simulink model "sig_kadet"  (R2024a)
settings: Solver=FixedStepAuto  StartTime=0.0  StopTime=10.0  FixedStep=framePeriod_s  RelTol=1e-3
undefined symbols (not defined in the file): Control, DiscIntNeverNeededParam, framePeriod_s
libraries: aerolibconvert2 x7, slpidlib x6
(part 1 of 2)
settings Model: Creator=brian  LastModifiedBy=zchen
settings SolverCC: AlgebraicLoopSolver=TrustRegion
settings OptimizationCC: DefaultParameterBehavior=Inlined  GainParamInheritBuiltInType=on  UseFloatMulNetSlope=on  DefaultUnderspecifiedDataType=single  InlineInvariantSignals=on  PassReuseOutputArgsAs=Individual arguments  ZeroExternalMemoryAtStartup=off  ZeroInternalMemoryAtStartup=off  NoFixptDivByZeroProtection=on  EfficientFloat2IntCast=on  LifeSpan=1  OptimizeBlockOrder=speed  DifferentSizesBufferReuse=on  EfficientTunableParamExpr=on
settings DebuggingCC: ParameterTunabilityLossMsg=error  UnconnectedInputMsg=warning  UnconnectedOutputMsg=warning  UnconnectedLineMsg=warning
settings HardwareCC: ProdBitPerPointer=32  ProdBitPerSizeT=32  ProdBitPerPtrDiffT=32  ProdLargestAtomicInteger=Long  ProdLargestAtomicFloat=Double  ProdWordSize=32  ProdLongLongMode=on  ProdHWDeviceType=NXP->Cortex-M4
settings ModelReferenceCC: EnableRefExpFcnMdlSchedulingChecks=on  ModelReferenceNumInstancesAllowed=Single
settings SFSimCC: SimParseCustomCode=off  MATLABDynamicMemAlloc=off
settings RTWCC: Description=Embedded Coder  SystemTargetFile=ert.tlc  GenCodeOnly=on  TemplateMakefile=ert_default_tmf  RTWVerbose=off  BuildConfiguration=Faster Runs  TargetLang=C++  GPUComputeCapability=3.5  DLArmComputeVersion=19.05
settings CodeAppCC: ForceParamTrailComments=on  IgnoreCustomStorageClasses=off  OperatorAnnotations=on  SimulinkDataObjDesc=on  SFDataObjDesc=on  CustomSymbolStrGlobalVar=rt$N$M  CustomSymbolStrType=$N$M  CustomSymbolStrFcn=$N$M$F  CustomSymbolStrMacro=$N$M  InsertBlockDesc=on
settings ERTTargetCC: TargetLangStandard=C++03 (ISO)  IncludeMdlTerminateFcn=off  CombineSignalStateStructs=on  SuppressErrorStatus=on  SupportAbsoluteTime=off  CodeInterfacePackaging=C++ class  SupportNonFinite=off  SupportComplex=off  ERTHeaderFileRootName=autocode$E  ERTSourceFileRootName=autocode$E  InlinedParameterPlacement=NonHierarchical  RootIOFormat=Structure reference  ERTCustomFileTemplate=example_file_process.tlc  ERTFilePackagingFormat=Compact  ArrayContainerType=std::array

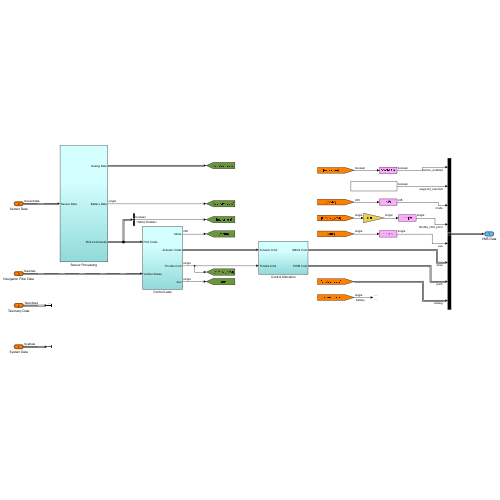
[thumbnail: Simulink's stored preview of the top-level diagram]
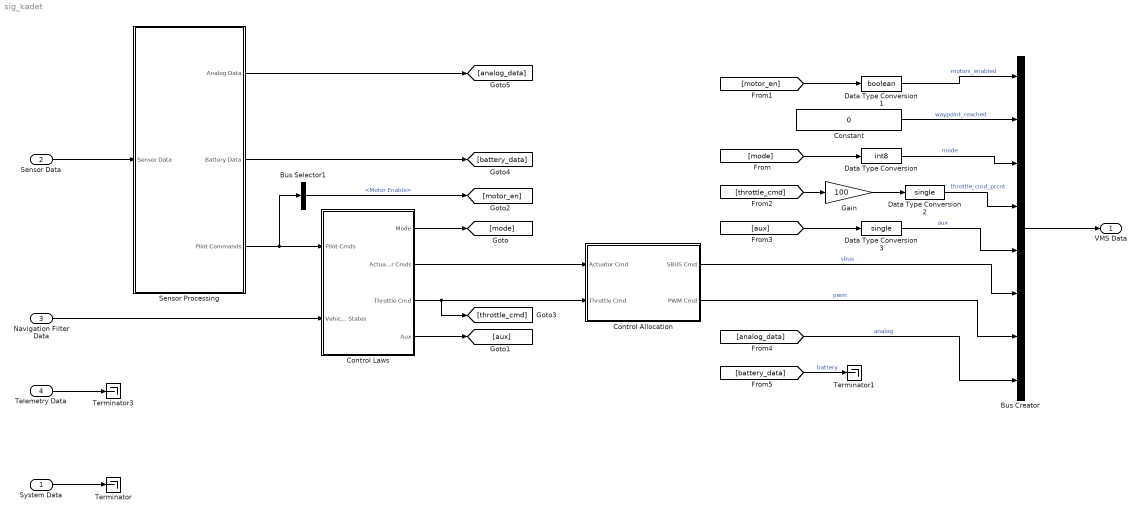
== system sig_kadet ==
  System Data : Inport  OutDataTypeStr=Bus: SysData  SampleTime=framePeriod_s  BusOutputAsStruct=on
  Sensor Data : Inport  Port=2  OutDataTypeStr=Bus: SensorData  SampleTime=framePeriod_s  BusOutputAsStruct=on
  Navigation Filter Data : Inport  Port=3  OutDataTypeStr=Bus: NavData  SampleTime=framePeriod_s  BusOutputAsStruct=on
  Telemetry Data : Inport  Port=4  OutDataTypeStr=Bus: TelemData  SampleTime=framePeriod_s  BusOutputAsStruct=on
  Bus Creator : BusCreator  Inputs=8
  Bus Selector1 : BusSelector  OutputSignals=Motor Enable
  Constant : Constant  Value=0  OutDataTypeStr=boolean
  Control Allocation : Subsystem
  Control Laws : Subsystem
  Data Type Conversion : DataTypeConversion  OutDataTypeStr=int8  SaturateOnIntegerOverflow=off  RndMeth=Floor
  Data Type Conversion1 : DataTypeConversion  OutDataTypeStr=boolean  SaturateOnIntegerOverflow=off  RndMeth=Floor
  Data Type Conversion2 : DataTypeConversion  OutDataTypeStr=single  SaturateOnIntegerOverflow=off  RndMeth=Floor
  Data Type Conversion3 : DataTypeConversion  OutDataTypeStr=single  SaturateOnIntegerOverflow=off  RndMeth=Floor
  Gain : Gain  Gain=100  OutDataTypeStr=single
  Sensor Processing : Subsystem
  Terminator : Terminator
  Terminator1 : Terminator
  Terminator3 : Terminator
  VMS Data : Outport  OutDataTypeStr=Bus: VmsData  SampleTime=framePeriod_s  BusOutputAsStruct=on
  wires:
  System Data/1 -> Terminator/1
  Sensor Data/1 -> Sensor Processing/1(Sensor Data)
  Telemetry Data/1 -> Terminator3/1
  Navigation Filter Data/1 -> Control Laws/2(Vehicle States)
  Control Laws/1(Mode) -> [mode]
  Control Laws/4(Aux) -> [aux]
  [mode] -> Data Type Conversion/1
  Data Type Conversion/1 -> Bus Creator/3  "mode"
  Bus Selector1/1 -> [motor_en]  "<Motor Enable>"
  [motor_en] -> Data Type Conversion1/1
  Data Type Conversion1/1 -> Bus Creator/1  "motors_enabled"
  Constant/1 -> Bus Creator/2  "waypoint_reached"
  Control Laws/3(Throttle Cmd) -> Control Allocation/2(Throttle Cmd), [throttle_cmd]
  [throttle_cmd] -> Gain/1
  Gain/1 -> Data Type Conversion2/1
  Data Type Conversion2/1 -> Bus Creator/4  "throttle_cmd_prcnt"
  [aux] -> Data Type Conversion3/1
  Data Type Conversion3/1 -> Bus Creator/5  "aux"
  Bus Creator/1 -> VMS Data/1
  Sensor Processing/3(Pilot Commands) -> Bus Selector1/1, Control Laws/1(Pilot Cmds)
  Sensor Processing/2(Battery Data) -> [battery_data]
  Sensor Processing/1(Analog Data) -> [analog_data]
  [analog_data] -> Bus Creator/8  "analog"
  Control Laws/2(Actuator Cmds) -> Control Allocation/1(Actuator Cmd)
  Control Allocation/1(SBUS Cmd) -> Bus Creator/6  "sbus"
  Control Allocation/2(PWM Cmd) -> Bus Creator/7  "pwm"
  [battery_data] -> Terminator1/1  "battery"

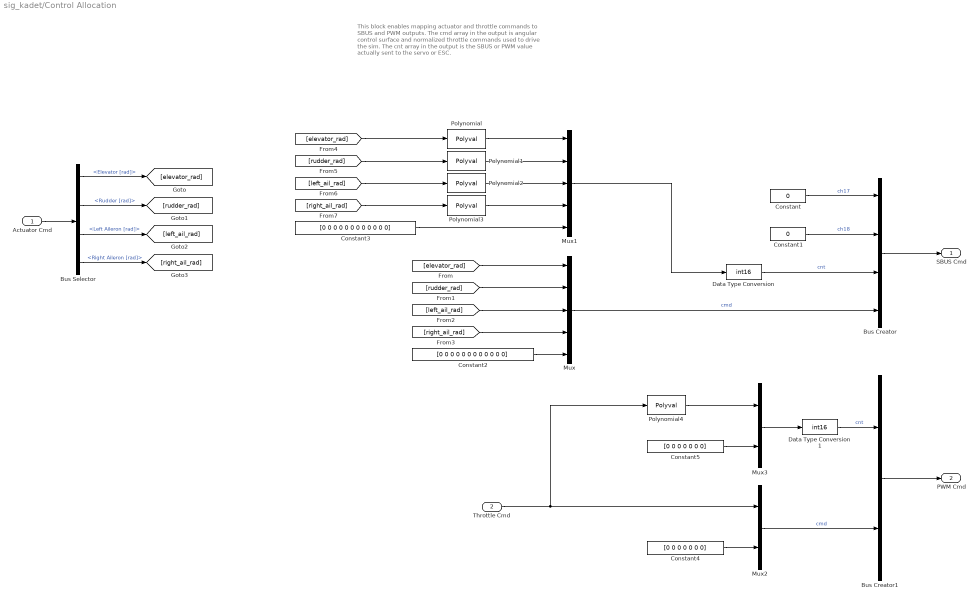
== system sig_kadet/Control Allocation ==
  note: This block enables mapping actuator and throttle commands
      | to SBUS and PWM outputs. The cmd array in the output
      | is angular control surface and normalized throttle commands
      | used to drive the sim. The cnt array in the output is the SBUS
      | or PWM value actually sent to the servo or ESC.
  Actuator Cmd : Inport
  Throttle Cmd : Inport  Port=2
  Bus Creator : BusCreator  Inputs=4
  Bus Creator1 : BusCreator  Inputs=2
  Bus Selector : BusSelector  OutputSignals=Elevator [rad],Rudder [rad],Left Aileron [rad],Right Aileron [rad]
  Constant : Constant  Value=0  OutDataTypeStr=boolean
  Constant1 : Constant  Value=0  OutDataTypeStr=boolean
  Constant2 : Constant  Value=[0 0 0 0 0 0 0 0 0 0 0 0]  OutDataTypeStr=single
  Constant3 : Constant  Value=[0 0 0 0 0 0 0 0 0 0 0 0]  OutDataTypeStr=single
  Constant4 : Constant  Value=[0 0 0 0 0 0 0]  OutDataTypeStr=single
  Constant5 : Constant  Value=[0 0 0 0 0 0 0]  OutDataTypeStr=single
  Data Type Conversion : DataTypeConversion  OutDataTypeStr=int16  SaturateOnIntegerOverflow=off  RndMeth=Floor
  Data Type Conversion1 : DataTypeConversion  OutDataTypeStr=int16  SaturateOnIntegerOverflow=off  RndMeth=Floor
  Mux : Mux  Inputs=5
  Mux1 : Mux  Inputs=5
  Mux2 : Mux  Inputs=2
  Mux3 : Mux  Inputs=2
  Polynomial : Polyval  Coefs=[1144.32190165984, 167.225360182927, 1558.74885501875, 1026.6382652891]
  Polynomial1 : Polyval  Coefs=[-930.322085258545, 148.612787752928, -1476.11502090935, 1006.01614399429]
  Polynomial2 : Polyval  Coefs=[1097.27825386315, 173.191562145482, 1642.60230905023, 1054.30469578325]
  Polynomial3 : Polyval  Coefs=[930.582953971947, 132.665450728095, 1620.14796233637, 1011.10438715363]
  Polynomial4 : Polyval  Coefs=[1000, 1000]
  SBUS Cmd : Outport
  PWM Cmd : Outport  Port=2
  wires:
  Constant/1 -> Bus Creator/1  "ch17"
  Constant1/1 -> Bus Creator/2  "ch18"
  Bus Creator/1 -> SBUS Cmd/1
  Mux/1 -> Bus Creator/4  "cmd"
  Mux1/1 -> Data Type Conversion/1
  Actuator Cmd/1 -> Bus Selector/1
  Bus Selector/1 -> [elevator_rad]  "<Elevator [rad]>"
  Bus Selector/2 -> [rudder_rad]  "<Rudder [rad]>"
  Bus Selector/3 -> [left_ail_rad]  "<Left Aileron [rad]>"
  Bus Selector/4 -> [right_ail_rad]  "<Right Aileron [rad]>"
  [elevator_rad] -> Mux/1
  [rudder_rad] -> Mux/2
  [left_ail_rad] -> Mux/3
  [right_ail_rad] -> Mux/4
  Constant2/1 -> Mux/5
  Constant3/1 -> Mux1/5
  [right_ail_rad] -> Polynomial3/1
  [left_ail_rad] -> Polynomial2/1
  [rudder_rad] -> Polynomial1/1
  [elevator_rad] -> Polynomial/1
  Data Type Conversion/1 -> Bus Creator/3  "cnt"
  Polynomial/1 -> Mux1/1
  Polynomial1/1 -> Mux1/2
  Polynomial2/1 -> Mux1/3
  Polynomial3/1 -> Mux1/4
  Bus Creator1/1 -> PWM Cmd/1
  Mux2/1 -> Bus Creator1/2  "cmd"
  Constant4/1 -> Mux2/2
  Throttle Cmd/1 -> Polynomial4/1, Mux2/1
  Polynomial4/1 -> Mux3/1
  Constant5/1 -> Mux3/2
  Mux3/1 -> Data Type Conversion1/1
  Data Type Conversion1/1 -> Bus Creator1/1  "cnt"

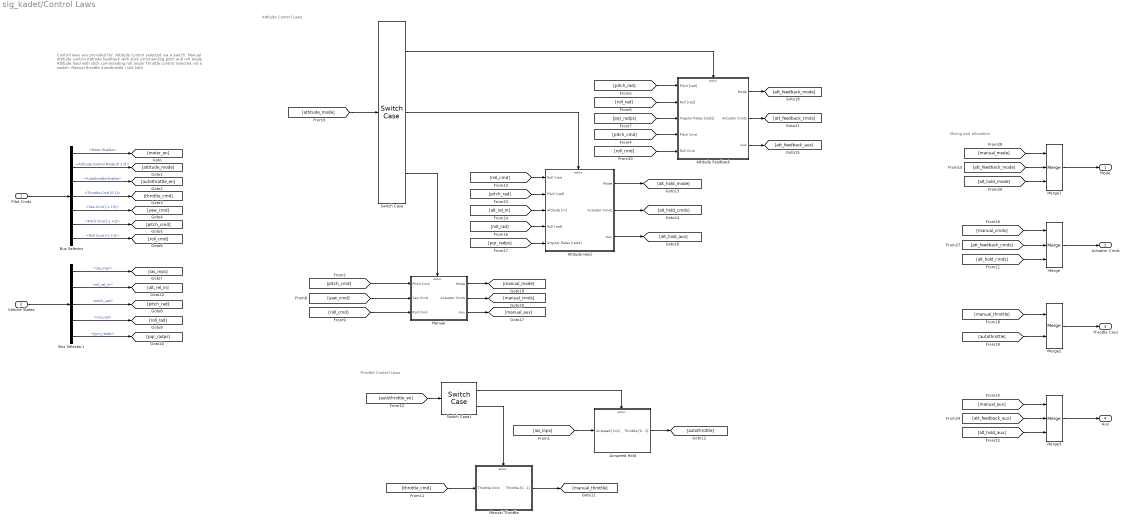
== system sig_kadet/Control Laws ==
  note: Control laws are provided for:
      | Attitude control selected via a switch:
      | Manual attitude control
      | Attitude feedback with stick commanding pitch and roll angle
      | Altitude hold with stick commanding roll angle
      | Throttle control selected via a switch:
      | Manual throttle
      | Autothrottle / IAS hold
  note: Throttle Control Laws
  note: Attitude Control Laws
  note: Mixing and Allocation
  Pilot Cmds : Inport
  Vehicle States : Inport  Port=2
  Airspeed Hold : Subsystem  TreatAsAtomicUnit=on
  Altitude Hold : Subsystem  TreatAsAtomicUnit=on
  Attitude Feedback : Subsystem  TreatAsAtomicUnit=on
  Bus Selector : BusSelector  OutputSignals=Motor Enable,Attitude Control Mode [0 1 2],Autothrottle Enable,Throttle Cmd [0 1],Yaw Cmd [-1 +1],Pitch Cmd [-1 +1],Roll Cmd [-1 +1]
  Bus Selector1 : BusSelector  OutputSignals=ias_mps,alt_rel_m,pitch_rad,roll_rad,gyro_radps
  Manual : Subsystem  TreatAsAtomicUnit=on
  Manual Throttle : Subsystem  TreatAsAtomicUnit=on
  Merge : Merge  Inputs=3
  Merge1 : Merge  Inputs=3
  Merge2 : Merge
  Merge3 : Merge  Inputs=3
  Switch Case : SwitchCase  CaseConditions={1, 2}
  Switch Case1 : SwitchCase
  Mode : Outport
  Actuator Cmds : Outport  Port=2
  Throttle Cmd : Outport  Port=3
  Aux : Outport  Port=4
  wires:
  Pilot Cmds/1 -> Bus Selector/1
  Bus Selector/1 -> [motor_en]  "<Motor Enable>"
  Bus Selector/2 -> [attitude_mode]  "<Attitude Control Mode [0 1 2]>"
  Bus Selector/3 -> [autothrottle_en]  "<Autothrottle Enable>"
  Bus Selector/4 -> [throttle_cmd]  "<Throttle Cmd [0 1]>"
  Bus Selector/5 -> [yaw_cmd]  "<Yaw Cmd [-1 +1]>"
  Bus Selector/6 -> [pitch_cmd]  "<Pitch Cmd [-1 +1]>"
  Bus Selector/7 -> [roll_cmd]  "<Roll Cmd [-1 +1]>"
  Vehicle States/1 -> Bus Selector1/1
  Bus Selector1/1 -> [ias_mps]  "<ias_mps>"
  Bus Selector1/3 -> [pitch_rad]  "<pitch_rad>"
  Bus Selector1/4 -> [roll_rad]  "<roll_rad>"
  Bus Selector1/5 -> [pqr_radps]  "<gyro_radps>"
  Airspeed Hold/1(Throttle [0 - 1]) -> [autothrottle]
  [ias_mps] -> Airspeed Hold/1(Airspeed [m/s])
  [autothrottle_en] -> Switch Case1/1
  [throttle_cmd] -> Manual Throttle/1(Throttle Cmd)
  Switch Case1/1 -> Airspeed Hold/Action
  Switch Case1/2 -> Manual Throttle/Action
  Manual Throttle/1(Throttle [0 - 1]) -> [manual_throttle]
  Manual/1(Mode) -> [manual_mode]
  [pqr_radps] -> Attitude Feedback/3(Angular Rates [rad/s])
  [pqr_radps] -> Altitude Hold/5(Angular Rates [rad/s])
  Altitude Hold/3(Aux) -> [alt_hold_aux]
  Altitude Hold/1(Mode) -> [alt_hold_mode]
  Manual/3(Aux) -> [manual_aux]
  [roll_cmd] -> Altitude Hold/1(Roll Cmd)
  Attitude Feedback/2(Actuator Cmds) -> [att_feedback_cmds]
  Switch Case/3 -> Manual/Action
  Manual/2(Actuator Cmds) -> [manual_cmds]
  Attitude Feedback/1(Mode) -> [att_feedback_mode]
  [roll_rad] -> Attitude Feedback/2(Roll [rad])
  [pitch_rad] -> Attitude Feedback/1(Pitch [rad])
  [alt_rel_m] -> Altitude Hold/3(Altitude [m])
  Switch Case/1 -> Attitude Feedback/Action
  Altitude Hold/2(Actuator Cmds) -> [alt_hold_cmds]
  [roll_rad] -> Altitude Hold/4(Roll [rad])
  [pitch_rad] -> Altitude Hold/2(Pitch [rad])
  Attitude Feedback/3(Aux) -> [att_feedback_aux]
  Switch Case/2 -> Altitude Hold/Action
  [attitude_mode] -> Switch Case/1
  [pitch_cmd] -> Manual/1(Pitch Cmd)
  [yaw_cmd] -> Manual/2(Yaw Cmd)
  [roll_cmd] -> Manual/3(Roll Cmd)
  [pitch_cmd] -> Attitude Feedback/4(Pitch Cmd)
  [roll_cmd] -> Attitude Feedback/5(Roll Cmd)
  Bus Selector1/2 -> [alt_rel_m]  "<alt_rel_m>"
  Merge3/1 -> Aux/1
  [att_feedback_aux] -> Merge3/2
  [alt_hold_aux] -> Merge3/3
  [manual_aux] -> Merge3/1
  [att_feedback_cmds] -> Merge/2
  [alt_hold_cmds] -> Merge/3
  [alt_hold_mode] -> Merge1/3
  Merge2/1 -> Throttle Cmd/1
  [manual_throttle] -> Merge2/1
  Merge1/1 -> Mode/1
  [manual_mode] -> Merge1/1
  [manual_cmds] -> Merge/1
  [att_feedback_mode] -> Merge1/2
  Merge/1 -> Actuator Cmds/1
  [autothrottle] -> Merge2/2

== system sig_kadet/Sensor Processing ==
  Sensor Data : Inport
  Analog Input Mapping : Subsystem
  Battery Data and State Estimation : Subsystem  Commented=on
  Bus Selector : BusSelector  OutputSignals=inceptor,adc
  Ground : Ground
  Pilot Stick Mapping : Subsystem
  Analog Data : Outport
  Battery Data : Outport  Port=2
  Pilot Commands : Outport  Port=3
  wires:
  Pilot Stick Mapping/1(Pilot Commands) -> Pilot Commands/1
  Sensor Data/1 -> Bus Selector/1
  Bus Selector/1 -> Pilot Stick Mapping/1(Inceptors)  "<inceptor>"
  Bus Selector/2 -> Analog Input Mapping/1(ADC)  "<adc>"
  Analog Input Mapping/1(Analog Data) -> Analog Data/1
  Ground/1 -> Battery Data/1

== system sig_kadet/Control Laws/Airspeed Hold ==
  Airspeed [m/s] : Inport
  Action Port : ActionPort  InitializeStates=reset  ActionPortLabel=case [ 1 ]:
  Constant1 : Constant  Value=Control.Airspeed.ref_mps  OutDataTypeStr=single
  Constant2 : Constant  Value=framePeriod_s  OutDataTypeStr=single
  PID Controller : slpidlib/PID Controller  Controller=PID  Form=Parallel  TimeDomain=Discrete-time  UseExternalTs=on  SampleTime=-1  IntegratorMethod=Forward Euler  FilterMethod=Forward Euler  ControllerParametersSource=internal  P=Control.Airspeed.p  I=Control.Airspeed.i  UseKiTs=off  D=0  UseExternalDerivativeSource=off  N=100  UseFilter=off  TunerSelectOption=Transfer Function Based (PID Tuner App)  ZeroCross=off  InitialConditionSource=internal  InitialConditionForIntegrator=0  InitialConditionForFilter=0  DifferentiatorICPrevScaledInput=0  ExternalReset=none  TrackingMode=off  Kt=1  LimitOutput=on  SatLimitsSource=internal  UpperSaturationLimit=Control.pla_lim_max  LowerSaturationLimit=Control.pla_lim_min  LinearizeAsGain=on  AntiWindupMode=clamping  Kb=1  LimitIntegrator=off  UpperIntegratorSaturationLimit=inf  LowerIntegratorSaturationLimit=-inf  PGainOutDataTypeStr=single  PProdOutDataTypeStr=single  POutMin=[]  POutMax=[]  IGainOutDataTypeStr=single  IProdOutDataTypeStr=single  IOutMin=[]  IOutMax=[]  DGainOutDataTypeStr=single  DProdOutDataTypeStr=single  DOutMin=[]  DOutMax=[]  NOutMin=[]  NOutMax=[]  SumOutDataTypeStr=single  SumOutMin=[]  SumOutMax=[]  SaturationOutDataTypeStr=single  SaturationOutMin=[]  SaturationOutMax=[]  PParamMin=[]  PParamMax=[]  IParamMin=[]  IParamMax=[]  DParamMin=[]  DParamMax=[]  NParamMin=[]  NParamMax=[]  KbParamMin=[]  KbParamMax=[]  KtParamMin=[]  KtParamMax=[]  KbOutMin=[]  KbOutMax=[]  KtOutMin=[]  KtOutMax=[]  IntegratorOutMin=[]  IntegratorOutMax=[]  FilterOutMin=[]  FilterOutMax=[]  SumI1OutMin=[]  SumI1OutMax=[]  SumI2OutMin=[]  SumI2OutMax=[]  SumI3OutMin=[]  SumI3OutMax=[]  SumI4OutMin=[]  SumI4OutMax=[]  SumDOutMin=[]  SumDOutMax=[]  DifferentiatorOutMin=[]  DifferentiatorOutMax=[]  FilterDiffOutCoefMin=[]  FilterDiffOutCoefMax=[]  ReciprocalOutMin=[]  ReciprocalOutMax=[]  SumDenOutMin=[]  SumDenOutMax=[]  SumNumOutMin=[]  SumNumOutMax=[]  DivideOutMin=[]  DivideOutMax=[]  UdiffTsProdOutMin=[]  UdiffTsProdOutMax=[]  NTsProdOutMin=[]  NTsProdOutMax=[]  UintegralTsProdOutMin=[]  UintegralTsProdOutMax=[]  UngainTsProdOutMin=[]  UngainTsProdOutMax=[]  ClampingZeroOutDataTypeStr=Inherit: Inherit via back propagation  ClampingZeroOutMin=[]  ClampingZeroOutMax=[]  FilterDenConstantOutDataTypeStr=Inherit: Inherit via back propagation  FilterDenConstantOutMin=[]  FilterDenConstantOutMax=[]  PCopyOutDataTypeStr=Inherit: Inherit via back propagation  PCopyOutMin=[]  PCopyOutMax=[]  NCopyOutDataTypeStr=Inherit: Inherit via back propagation  NCopyOutMin=[]  NCopyOutMax=[]  IntegratorContinuousStateAttributes=''  IntegratorStateMustResolveToSignalObject=off  IntegratorRTWStateStorageClass=Auto  FilterContinuousStateAttributes=''  FilterStateMustResolveToSignalObject=off  FilterRTWStateStorageClass=Auto  ParallelPVariant=InternalParameters  IdealPVariant=Disabled  IVariant=InternalParameters  DVariant=InternalParameters  IntegratorVariant=Discrete  SatVariant=Enabled  AWVariant=DiscClampingParallel  PCopyVariant=Disabled  TRVariant=Disabled  FdbkBlocksVariant=Forward  IdealPFdbkVariant=Disabled  SatFdbkVariant=Disabled  DerivativeFilterVariant=Differentiator  NVariant=Passthrough  NCopyVariant=Disabled_SignalSpec  FilterICVariant=InternalICsDifferentiator  IntegratorICVariant=InternalICs  ExternalResetVariant=Disabled  TRSumVariant=Passthrough  SumFdbkVariant=Disabled  SumVariant=Sum_PID  TsampFilterVariant=ExternalTs  TsampNgainVariant=Passthrough  TsampIntegralVariant=ExternalTs  ExternalSaturationOutDataTypeStr=Inherit: Same as second input  DerivativeSourceVariant=ErrorSignal
  Subtract : Sum  Inputs=+-  AccumDataTypeStr=single
  Throttle [0 - 1] : Outport
  wires:
  PID Controller/1 -> Throttle [0 - 1]/1  "Throttle [0 - 1]"
  Subtract/1 -> PID Controller/1
  Constant2/1 -> PID Controller/2
  Airspeed [m/s]/1 -> Subtract/2
  Constant1/1 -> Subtract/1

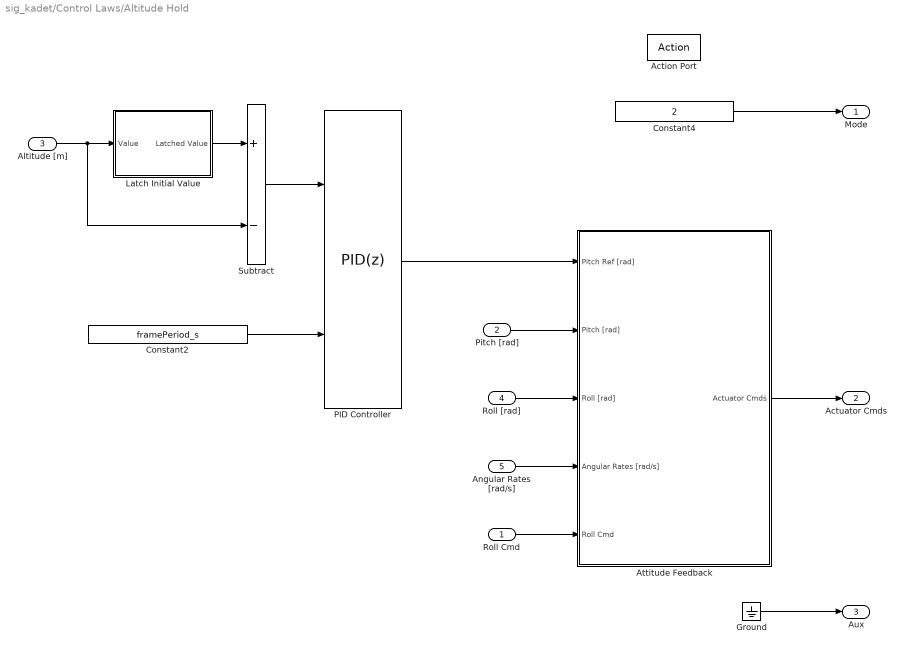
== system sig_kadet/Control Laws/Altitude Hold ==
  Roll Cmd : Inport
  Pitch [rad] : Inport  Port=2
  Altitude [m] : Inport  Port=3
  Roll [rad] : Inport  Port=4
  Angular Rates [rad/s] : Inport  Port=5
  Action Port : ActionPort  InitializeStates=reset  ActionPortLabel=case [ 2 ]:
  Attitude Feedback : Subsystem  TreatAsAtomicUnit=on
  Constant2 : Constant  Value=framePeriod_s  OutDataTypeStr=single
  Constant4 : Constant  Value=2  OutDataTypeStr=int8
  Ground : Ground
  Latch Initial Value : Subsystem
  PID Controller : slpidlib/PID Controller  Controller=PID  Form=Parallel  TimeDomain=Discrete-time  UseExternalTs=on  SampleTime=-1  IntegratorMethod=Forward Euler  FilterMethod=Forward Euler  ControllerParametersSource=internal  P=Control.Altitude.p  I=Control.Altitude.i  UseKiTs=off  D=0  UseExternalDerivativeSource=off  N=100  UseFilter=off  TunerSelectOption=Transfer Function Based (PID Tuner App)  ZeroCross=off  InitialConditionSource=internal  InitialConditionForIntegrator=0  InitialConditionForFilter=0  DifferentiatorICPrevScaledInput=0  ExternalReset=none  TrackingMode=off  Kt=1  LimitOutput=on  SatLimitsSource=internal  UpperSaturationLimit=deg2rad(Control.pitch_lim_deg)  LowerSaturationLimit=-deg2rad(Control.pitch_lim_deg)  LinearizeAsGain=on  AntiWindupMode=clamping  Kb=1  LimitIntegrator=off  UpperIntegratorSaturationLimit=inf  LowerIntegratorSaturationLimit=-inf  PGainOutDataTypeStr=single  PProdOutDataTypeStr=single  POutMin=[]  POutMax=[]  IGainOutDataTypeStr=single  IProdOutDataTypeStr=single  IOutMin=[]  IOutMax=[]  DGainOutDataTypeStr=single  DProdOutDataTypeStr=single  DOutMin=[]  DOutMax=[]  NOutMin=[]  NOutMax=[]  SumOutDataTypeStr=single  SumOutMin=[]  SumOutMax=[]  SaturationOutDataTypeStr=single  SaturationOutMin=[]  SaturationOutMax=[]  PParamMin=[]  PParamMax=[]  IParamMin=[]  IParamMax=[]  DParamMin=[]  DParamMax=[]  NParamMin=[]  NParamMax=[]  KbParamMin=[]  KbParamMax=[]  KtParamMin=[]  KtParamMax=[]  KbOutMin=[]  KbOutMax=[]  KtOutMin=[]  KtOutMax=[]  IntegratorOutMin=[]  IntegratorOutMax=[]  FilterOutMin=[]  FilterOutMax=[]  SumI1OutMin=[]  SumI1OutMax=[]  SumI2OutMin=[]  SumI2OutMax=[]  SumI3OutMin=[]  SumI3OutMax=[]  SumI4OutMin=[]  SumI4OutMax=[]  SumDOutMin=[]  SumDOutMax=[]  DifferentiatorOutMin=[]  DifferentiatorOutMax=[]  FilterDiffOutCoefMin=[]  FilterDiffOutCoefMax=[]  ReciprocalOutMin=[]  ReciprocalOutMax=[]  SumDenOutMin=[]  SumDenOutMax=[]  SumNumOutMin=[]  SumNumOutMax=[]  DivideOutMin=[]  DivideOutMax=[]  UdiffTsProdOutMin=[]  UdiffTsProdOutMax=[]  NTsProdOutMin=[]  NTsProdOutMax=[]  UintegralTsProdOutMin=[]  UintegralTsProdOutMax=[]  UngainTsProdOutMin=[]  UngainTsProdOutMax=[]  ClampingZeroOutDataTypeStr=Inherit: Inherit via back propagation  ClampingZeroOutMin=[]  ClampingZeroOutMax=[]  FilterDenConstantOutDataTypeStr=Inherit: Inherit via back propagation  FilterDenConstantOutMin=[]  FilterDenConstantOutMax=[]  PCopyOutDataTypeStr=Inherit: Inherit via back propagation  PCopyOutMin=[]  PCopyOutMax=[]  NCopyOutDataTypeStr=Inherit: Inherit via back propagation  NCopyOutMin=[]  NCopyOutMax=[]  IntegratorContinuousStateAttributes=''  IntegratorStateMustResolveToSignalObject=off  IntegratorRTWStateStorageClass=Auto  FilterContinuousStateAttributes=''  FilterStateMustResolveToSignalObject=off  FilterRTWStateStorageClass=Auto  ParallelPVariant=InternalParameters  IdealPVariant=Disabled  IVariant=InternalParameters  DVariant=InternalParameters  IntegratorVariant=Discrete  SatVariant=Enabled  AWVariant=DiscClampingParallel  PCopyVariant=Disabled  TRVariant=Disabled  FdbkBlocksVariant=Forward  IdealPFdbkVariant=Disabled  SatFdbkVariant=Disabled  DerivativeFilterVariant=Differentiator  NVariant=Passthrough  NCopyVariant=Disabled_SignalSpec  FilterICVariant=InternalICsDifferentiator  IntegratorICVariant=InternalICs  ExternalResetVariant=Disabled  TRSumVariant=Passthrough  SumFdbkVariant=Disabled  SumVariant=Sum_PID  TsampFilterVariant=ExternalTs  TsampNgainVariant=Passthrough  TsampIntegralVariant=ExternalTs  ExternalSaturationOutDataTypeStr=Inherit: Same as second input  DerivativeSourceVariant=ErrorSignal
  Subtract : Sum  Inputs=+-
  Mode : Outport
  Actuator Cmds : Outport  Port=2
  Aux : Outport  Port=3
  wires:
  Constant4/1 -> Mode/1
  Angular Rates [rad/s]/1 -> Attitude Feedback/4(Angular Rates [rad/s])
  Roll [rad]/1 -> Attitude Feedback/3(Roll [rad])
  Roll Cmd/1 -> Attitude Feedback/5(Roll Cmd)
  Attitude Feedback/1(Actuator Cmds) -> Actuator Cmds/1
  Altitude [m]/1 -> Subtract/2, Latch Initial Value/1(Value)
  Constant2/1 -> PID Controller/2
  Latch Initial Value/1(Latched Value) -> Subtract/1
  Subtract/1 -> PID Controller/1
  Ground/1 -> Aux/1
  Pitch [rad]/1 -> Attitude Feedback/2(Pitch [rad])
  PID Controller/1 -> Attitude Feedback/1(Pitch Ref [rad])

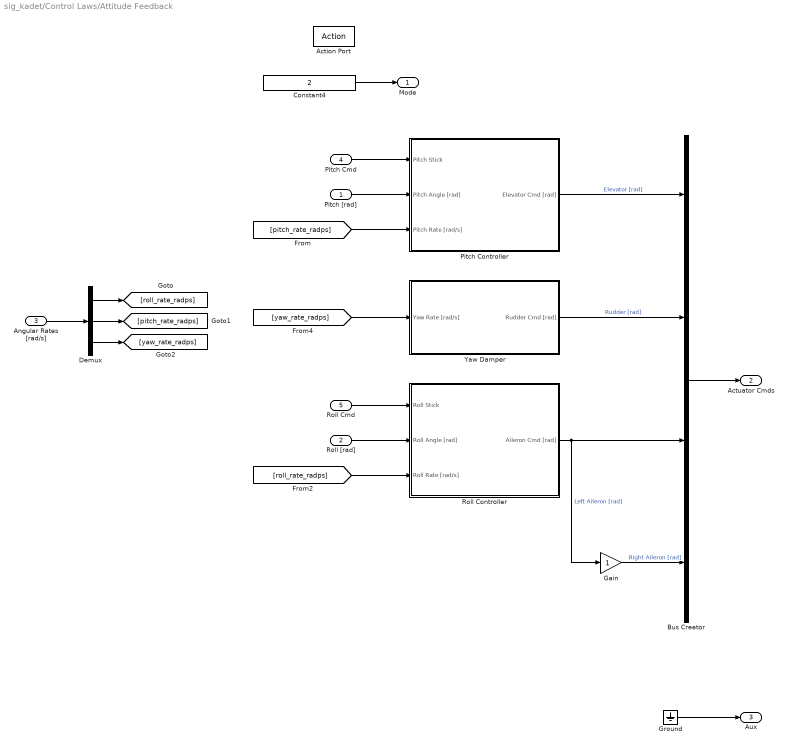
== system sig_kadet/Control Laws/Attitude Feedback ==
  Pitch [rad] : Inport
  Roll [rad] : Inport  Port=2
  Angular Rates [rad/s] : Inport  Port=3
  Pitch Cmd : Inport  Port=4
  Roll Cmd : Inport  Port=5
  Action Port : ActionPort  InitializeStates=reset  ActionPortLabel=case [ 1 ]:
  Bus Creator : BusCreator  Inputs=4
  Constant4 : Constant  Value=2  OutDataTypeStr=int8
  Demux : Demux  Outputs=3
  Gain : Gain
  Ground : Ground
  Pitch Controller : Subsystem
  Roll Controller : Subsystem
  Yaw Damper : Subsystem
  Mode : Outport
  Actuator Cmds : Outport  Port=2
  Aux : Outport  Port=3
  wires:
  Constant4/1 -> Mode/1
  Pitch [rad]/1 -> Pitch Controller/2(Pitch Angle [rad])
  Angular Rates [rad/s]/1 -> Demux/1
  Demux/1 -> [roll_rate_radps]
  Demux/3 -> [yaw_rate_radps]
  Demux/2 -> [pitch_rate_radps]
  [pitch_rate_radps] -> Pitch Controller/3(Pitch Rate [rad/s])
  Pitch Cmd/1 -> Pitch Controller/1(Pitch Stick)
  Pitch Controller/1(Elevator Cmd [rad]) -> Bus Creator/1  "Elevator [rad]"
  Bus Creator/1 -> Actuator Cmds/1
  Gain/1 -> Bus Creator/4  "Right Aileron [rad]"
  Roll Controller/1(Aileron Cmd [rad]) -> Gain/1, Bus Creator/3  "Left Aileron [rad]"
  Yaw Damper/1(Rudder Cmd [rad]) -> Bus Creator/2  "Rudder [rad]"
  Roll [rad]/1 -> Roll Controller/2(Roll Angle [rad])
  [roll_rate_radps] -> Roll Controller/3(Roll Rate [rad/s])
  Roll Cmd/1 -> Roll Controller/1(Roll Stick)
  [yaw_rate_radps] -> Yaw Damper/1(Yaw Rate [rad/s])
  Ground/1 -> Aux/1

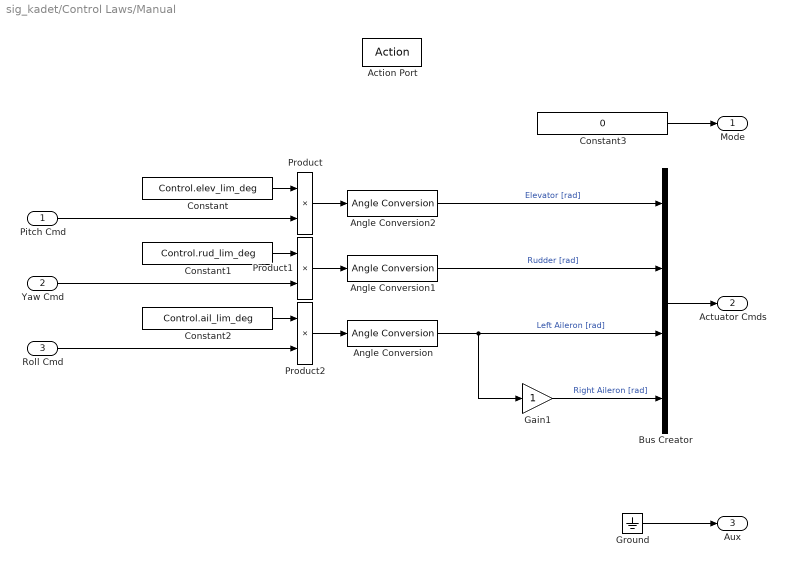
== system sig_kadet/Control Laws/Manual ==
  Pitch Cmd : Inport
  Yaw Cmd : Inport  Port=2
  Roll Cmd : Inport  Port=3
  Action Port : ActionPort  InitializeStates=reset  ActionPortLabel=default:
  Angle Conversion : aerolibconvert2/Angle Conversion  IU=deg  OU=rad
  Angle Conversion1 : aerolibconvert2/Angle Conversion  IU=deg  OU=rad
  Angle Conversion2 : aerolibconvert2/Angle Conversion  IU=deg  OU=rad
  Bus Creator : BusCreator  Inputs=4
  Constant : Constant  Value=Control.elev_lim_deg  OutDataTypeStr=single
  Constant1 : Constant  Value=Control.rud_lim_deg  OutDataTypeStr=single
  Constant2 : Constant  Value=Control.ail_lim_deg  OutDataTypeStr=single
  Constant3 : Constant  Value=0  OutDataTypeStr=int8
  Gain1 : Gain  OutDataTypeStr=single
  Ground : Ground
  Product : Product  OutDataTypeStr=single
  Product1 : Product  OutDataTypeStr=single
  Product2 : Product  OutDataTypeStr=single
  Mode : Outport
  Actuator Cmds : Outport  Port=2
  Aux : Outport  Port=3
  wires:
  Angle Conversion1/1 -> Bus Creator/2  "Rudder [rad]"
  Product2/1 -> Angle Conversion/1
  Yaw Cmd/1 -> Product1/2
  Roll Cmd/1 -> Product2/2
  Angle Conversion/1 -> Gain1/1, Bus Creator/3  "Left Aileron [rad]"
  Product1/1 -> Angle Conversion1/1
  Pitch Cmd/1 -> Product/2
  Gain1/1 -> Bus Creator/4  "Right Aileron [rad]"
  Constant1/1 -> Product1/1
  Angle Conversion2/1 -> Bus Creator/1  "Elevator [rad]"
  Product/1 -> Angle Conversion2/1
  Constant/1 -> Product/1
  Constant2/1 -> Product2/1
  Bus Creator/1 -> Actuator Cmds/1
  Constant3/1 -> Mode/1
  Ground/1 -> Aux/1

== system sig_kadet/Control Laws/Manual Throttle ==
  Throttle Cmd : Inport
  Action Port : ActionPort  InitializeStates=reset  ActionPortLabel=default:
  Gain : Gain  OutDataTypeStr=single
  Throttle [0 - 1] : Outport
  wires:
  Gain/1 -> Throttle [0 - 1]/1  "Throttle [0 - 1]"
  Throttle Cmd/1 -> Gain/1

== system sig_kadet/Sensor Processing/Analog Input Mapping ==
  note: FMU-R v2.x has 8 channels of analog input
      | data from 0 - 3.3V. The measured voltage
      | is available from the ADC data input, this is
      | an opportunity to map the voltage data to
      | engineering units (i.e. control surface position,
      | acceleration, etc) for logging and use elsewhere
      | in the VMS.
  ADC : Inport
  Bus Creator : BusCreator  Inputs=1  OutDataTypeStr=Bus: AnalogData
  Bus Selector : BusSelector  OutputSignals=volt
  Gain : Gain  Gain=0
  Analog Data : Outport
  wires:
  ADC/1 -> Bus Selector/1
  Bus Selector/1 -> Gain/1  "<volt>"
  Gain/1 -> Bus Creator/1  "val"
  Bus Creator/1 -> Analog Data/1

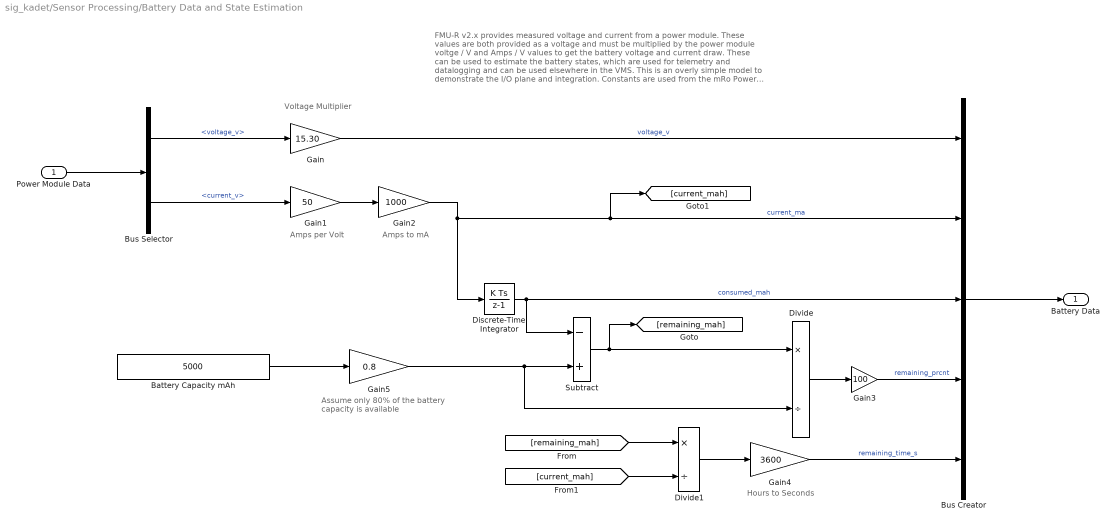
== system sig_kadet/Sensor Processing/Battery Data and State Estimation ==
  note: Assume only 80% of
      | the battery capacity is available
  note: Hours to Seconds
  note: Amps to mA
  note: Amps per Volt
  note: Voltage Multiplier
  note: FMU-R v2.x provides measured voltage and current from a power module.
      | These values are both provided as a voltage and must be multiplied by the
      | power module voltge / V and Amps / V values to get the battery voltage
      | and current draw. These can be used to estimate the battery states, which
      | are used for telemetry and datalogging and can be used elsewhere in the VMS.
      |
      | This is an overly simple model to demonstrate the I/O plane and integration.
      | Constants are used from the mRo Power Zero module.
  Power Module Data : Inport
  Battery Capacity mAh : Constant  Value=5000  OutDataTypeStr=single
  Bus Creator : BusCreator  Inputs=5  OutDataTypeStr=Bus: BatteryData
  Bus Selector : BusSelector  OutputSignals=voltage_v,current_v
  Discrete-Time Integrator : DiscreteIntegrator  SampleTime=framePeriod_s  ICPrevOutput=DiscIntNeverNeededParam  ICPrevScaledInput=DiscIntNeverNeededParam
  Divide : Product  Inputs=*/
  Divide1 : Product  Inputs=*/
  Gain : Gain  Gain=15.30
  Gain1 : Gain  Gain=50
  Gain2 : Gain  Gain=1000
  Gain3 : Gain  Gain=100
  Gain4 : Gain  Gain=3600
  Gain5 : Gain  Gain=0.8
  Subtract : Sum  Inputs=-+
  Battery Data : Outport
  wires:
  Power Module Data/1 -> Bus Selector/1
  Bus Selector/1 -> Gain/1  "<voltage_v>"
  Bus Selector/2 -> Gain1/1  "<current_v>"
  Gain1/1 -> Gain2/1
  Gain2/1 -> [current_mah], Bus Creator/2, Discrete-Time Integrator/1  "current_ma"
  Gain/1 -> Bus Creator/1  "voltage_v"
  Discrete-Time Integrator/1 -> Subtract/1, Bus Creator/3  "consumed_mah"
  Bus Creator/1 -> Battery Data/1
  Subtract/1 -> [remaining_mah], Divide/1
  Gain5/1 -> Divide/2, Subtract/2
  Divide/1 -> Gain3/1
  Gain3/1 -> Bus Creator/4  "remaining_prcnt"
  [remaining_mah] -> Divide1/1
  [current_mah] -> Divide1/2
  Gain4/1 -> Bus Creator/5  "remaining_time_s"
  Divide1/1 -> Gain4/1
  Battery Capacity mAh/1 -> Gain5/1

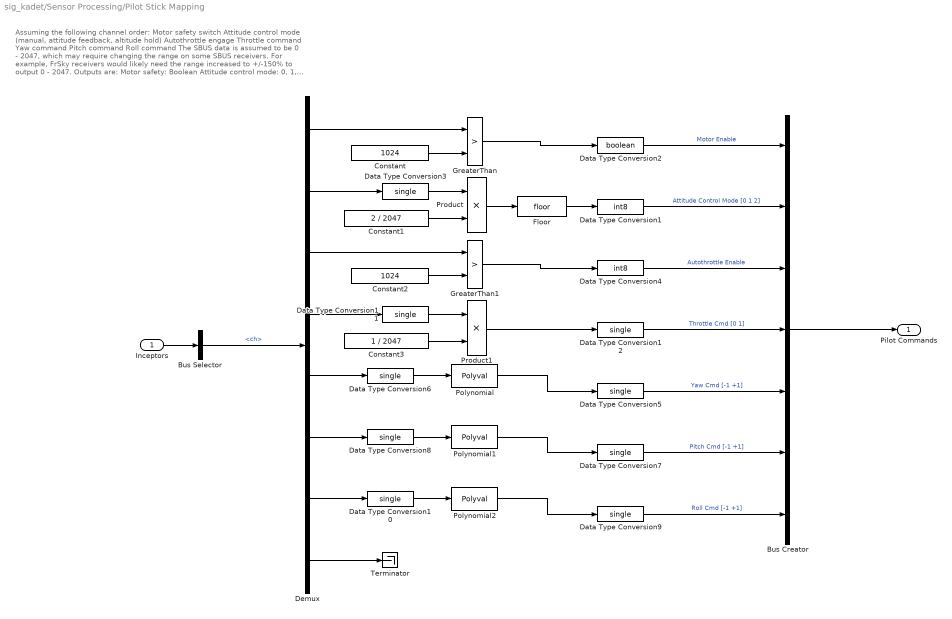
== system sig_kadet/Sensor Processing/Pilot Stick Mapping ==
  note: Assuming the following channel order:
      | Motor safety switch
      | Attitude control mode (manual, attitude feedback, altitude hold)
      | Autothrottle engage
      | Throttle command
      | Yaw command
      | Pitch command
      | Roll command
      |
      | The SBUS data is assumed to be 0 - 2047, which may require changing the
      | range on some SBUS receivers. For example, FrSky receivers would
      | likely need the range increased to +/-150% to output 0 - 2047.
      |
      | Outputs are:
      | Motor safety: Boolean
      | Attitude control mode: 0, 1, 2 integer
      | Autothrottle engage: Boolean
      | Throttle command: 0 to 1 single
      | Yaw command: -1 to +1 single
      | Pitch command: -1 to +1 single
      | Roll command: -1 to +1 single
  Inceptors : Inport
  Bus Creator : BusCreator  Inputs=7
  Bus Selector : BusSelector  OutputSignals=ch
  Constant : Constant  Value=1024
  Constant1 : Constant  Value=2 / 2047  OutDataTypeStr=single
  Constant2 : Constant  Value=1024  OutDataTypeStr=int16
  Constant3 : Constant  Value=1 / 2047  OutDataTypeStr=single
  Data Type Conversion1 : DataTypeConversion  OutDataTypeStr=int8  SaturateOnIntegerOverflow=off  RndMeth=Floor
  Data Type Conversion{3,5..12} (9 alike) : DataTypeConversion  OutDataTypeStr=single  SaturateOnIntegerOverflow=off  RndMeth=Floor
  Data Type Conversion2 : DataTypeConversion  OutDataTypeStr=boolean  SaturateOnIntegerOverflow=off  RndMeth=Floor
  Data Type Conversion4 : DataTypeConversion  OutDataTypeStr=int8  SaturateOnIntegerOverflow=off  RndMeth=Floor
  Demux : Demux  Outputs=[1 1 1 1 1 1 1 9]
  Floor : Rounding
  GreaterThan : RelationalOperator  Operator=>  OutDataTypeStr=boolean  RndMeth=Simplest  InputSameDT=off
  GreaterThan1 : RelationalOperator  Operator=>  OutDataTypeStr=boolean  RndMeth=Simplest  InputSameDT=off
  Polynomial : Polyval  Coefs=[2/2047 -1]
  Polynomial1 : Polyval  Coefs=[2/2047 -1]
  Polynomial2 : Polyval  Coefs=[2/2047 -1]
  Product : Product
  Product1 : Product
  Terminator : Terminator
  Pilot Commands : Outport
  wires:
  Inceptors/1 -> Bus Selector/1
  Bus Selector/1 -> Demux/1  "<ch>"
  Constant/1 -> GreaterThan/2
  Demux/1 -> GreaterThan/1
  GreaterThan/1 -> Data Type Conversion2/1
  Demux/2 -> Data Type Conversion3/1
  Product/1 -> Floor/1
  Constant1/1 -> Product/2
  Demux/3 -> GreaterThan1/1
  Constant2/1 -> GreaterThan1/2
  GreaterThan1/1 -> Data Type Conversion4/1
  Floor/1 -> Data Type Conversion1/1
  Data Type Conversion3/1 -> Product/1
  Data Type Conversion6/1 -> Polynomial/1
  Polynomial/1 -> Data Type Conversion5/1
  Polynomial1/1 -> Data Type Conversion7/1
  Data Type Conversion8/1 -> Polynomial1/1
  Demux/5 -> Data Type Conversion6/1
  Demux/6 -> Data Type Conversion8/1
  Data Type Conversion10/1 -> Polynomial2/1
  Polynomial2/1 -> Data Type Conversion9/1
  Demux/7 -> Data Type Conversion10/1
  Demux/8 -> Terminator/1
  Data Type Conversion11/1 -> Product1/1
  Constant3/1 -> Product1/2
  Demux/4 -> Data Type Conversion11/1
  Product1/1 -> Data Type Conversion12/1
  Bus Creator/1 -> Pilot Commands/1
  Data Type Conversion2/1 -> Bus Creator/1  "Motor Enable"
  Data Type Conversion1/1 -> Bus Creator/2  "Attitude Control Mode [0 1 2]"
  Data Type Conversion4/1 -> Bus Creator/3  "Autothrottle Enable"
  Data Type Conversion12/1 -> Bus Creator/4  "Throttle Cmd [0 1]"
  Data Type Conversion5/1 -> Bus Creator/5  "Yaw Cmd [-1 +1]"
  Data Type Conversion7/1 -> Bus Creator/6  "Pitch Cmd [-1 +1]"
  Data Type Conversion9/1 -> Bus Creator/7  "Roll Cmd [-1 +1]"

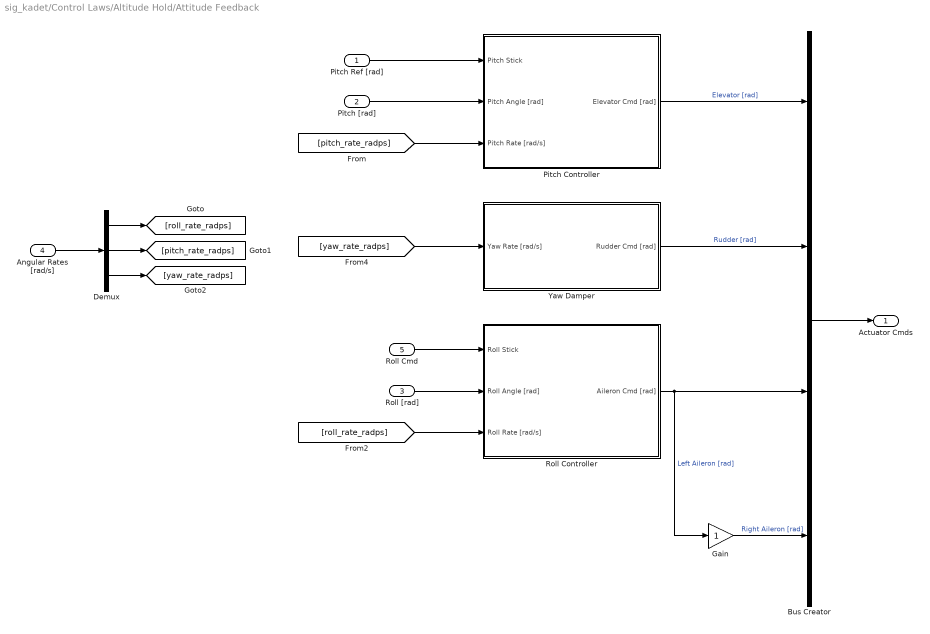
== system sig_kadet/Control Laws/Altitude Hold/Attitude Feedback ==
  Pitch Ref [rad] : Inport
  Pitch [rad] : Inport  Port=2
  Roll [rad] : Inport  Port=3
  Angular Rates [rad/s] : Inport  Port=4
  Roll Cmd : Inport  Port=5
  Bus Creator : BusCreator  Inputs=4
  Demux : Demux  Outputs=3
  Gain : Gain
  Pitch Controller : Subsystem
  Roll Controller : Subsystem
  Yaw Damper : Subsystem
  Actuator Cmds : Outport
  wires:
  Pitch [rad]/1 -> Pitch Controller/2(Pitch Angle [rad])
  Angular Rates [rad/s]/1 -> Demux/1
  Demux/1 -> [roll_rate_radps]
  Demux/3 -> [yaw_rate_radps]
  Demux/2 -> [pitch_rate_radps]
  [pitch_rate_radps] -> Pitch Controller/3(Pitch Rate [rad/s])
  Pitch Ref [rad]/1 -> Pitch Controller/1(Pitch Stick)
  Pitch Controller/1(Elevator Cmd [rad]) -> Bus Creator/1  "Elevator [rad]"
  Bus Creator/1 -> Actuator Cmds/1
  Gain/1 -> Bus Creator/4  "Right Aileron [rad]"
  Roll Controller/1(Aileron Cmd [rad]) -> Gain/1, Bus Creator/3  "Left Aileron [rad]"
  Yaw Damper/1(Rudder Cmd [rad]) -> Bus Creator/2  "Rudder [rad]"
  Roll [rad]/1 -> Roll Controller/2(Roll Angle [rad])
  [roll_rate_radps] -> Roll Controller/3(Roll Rate [rad/s])
  Roll Cmd/1 -> Roll Controller/1(Roll Stick)
  [yaw_rate_radps] -> Yaw Damper/1(Yaw Rate [rad/s])

== system sig_kadet/Control Laws/Altitude Hold/Latch Initial Value ==
  Value : Inport
  Constant : Constant  Value=0
  Switch : Switch  Criteria=u2 > Threshold  SaturateOnIntegerOverflow=off  InputSameDT=off
  Unit Delay : UnitDelay  SampleTime=-1  HasFrameUpgradeWarning=on
  Unit Delay1 : UnitDelay  InitialCondition=1  SampleTime=-1  HasFrameUpgradeWarning=on
  Latched Value : Outport
  wires:
  Unit Delay/1 -> Switch/3
  Value/1 -> Switch/1
  Constant/1 -> Unit Delay1/1
  Unit Delay1/1 -> Switch/2
  Switch/1 -> Unit Delay/1, Latched Value/1

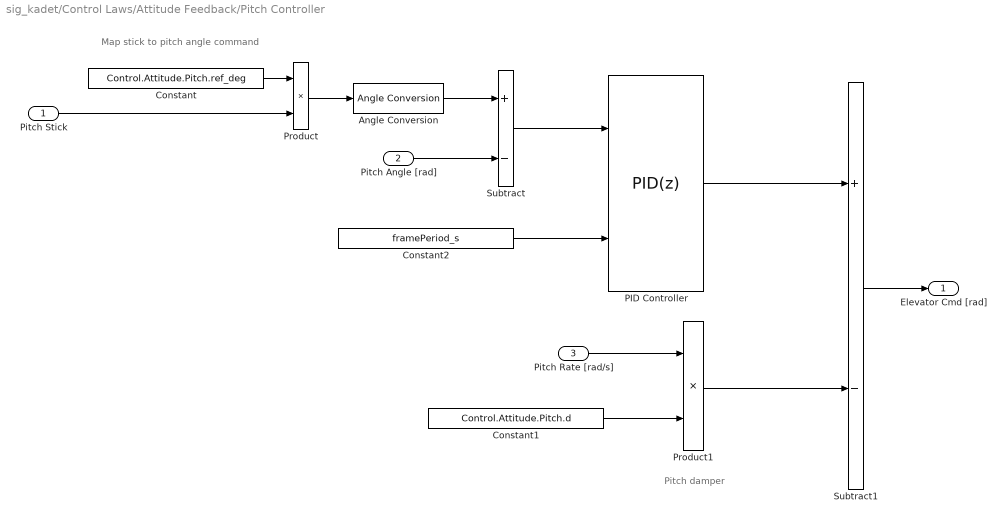
== system sig_kadet/Control Laws/Attitude Feedback/Pitch Controller ==
  note: Pitch damper
  note: Map stick to pitch angle command
  Pitch Stick : Inport
  Pitch Angle [rad] : Inport  Port=2
  Pitch Rate [rad/s] : Inport  Port=3
  Angle Conversion : aerolibconvert2/Angle Conversion  IU=deg  OU=rad
  Constant : Constant  Value=Control.Attitude.Pitch.ref_deg  OutDataTypeStr=single
  Constant1 : Constant  Value=Control.Attitude.Pitch.d  OutDataTypeStr=single
  Constant2 : Constant  Value=framePeriod_s  OutDataTypeStr=single
  PID Controller : slpidlib/PID Controller  Controller=PID  Form=Parallel  TimeDomain=Discrete-time  UseExternalTs=on  SampleTime=-1  IntegratorMethod=Forward Euler  FilterMethod=Forward Euler  ControllerParametersSource=internal  P=Control.Attitude.Pitch.p  I=Control.Attitude.Pitch.i  UseKiTs=off  D=0  UseExternalDerivativeSource=off  N=100  UseFilter=off  TunerSelectOption=Transfer Function Based (PID Tuner App)  ZeroCross=off  InitialConditionSource=internal  InitialConditionForIntegrator=0  InitialConditionForFilter=0  DifferentiatorICPrevScaledInput=0  ExternalReset=none  TrackingMode=off  Kt=1  LimitOutput=on  SatLimitsSource=internal  UpperSaturationLimit=deg2rad(Control.elev_lim_deg)  LowerSaturationLimit=-deg2rad(Control.elev_lim_deg)  LinearizeAsGain=on  AntiWindupMode=clamping  Kb=1  LimitIntegrator=off  UpperIntegratorSaturationLimit=inf  LowerIntegratorSaturationLimit=-inf  PGainOutDataTypeStr=single  PProdOutDataTypeStr=single  POutMin=[]  POutMax=[]  IGainOutDataTypeStr=single  IProdOutDataTypeStr=single  IOutMin=[]  IOutMax=[]  DGainOutDataTypeStr=single  DProdOutDataTypeStr=single  DOutMin=[]  DOutMax=[]  NOutMin=[]  NOutMax=[]  SumOutDataTypeStr=single  SumOutMin=[]  SumOutMax=[]  SaturationOutDataTypeStr=single  SaturationOutMin=[]  SaturationOutMax=[]  PParamMin=[]  PParamMax=[]  IParamMin=[]  IParamMax=[]  DParamMin=[]  DParamMax=[]  NParamMin=[]  NParamMax=[]  KbParamMin=[]  KbParamMax=[]  KtParamMin=[]  KtParamMax=[]  KbOutMin=[]  KbOutMax=[]  KtOutMin=[]  KtOutMax=[]  IntegratorOutMin=[]  IntegratorOutMax=[]  FilterOutMin=[]  FilterOutMax=[]  SumI1OutMin=[]  SumI1OutMax=[]  SumI2OutMin=[]  SumI2OutMax=[]  SumI3OutMin=[]  SumI3OutMax=[]  SumI4OutMin=[]  SumI4OutMax=[]  SumDOutMin=[]  SumDOutMax=[]  DifferentiatorOutMin=[]  DifferentiatorOutMax=[]  FilterDiffOutCoefMin=[]  FilterDiffOutCoefMax=[]  ReciprocalOutMin=[]  ReciprocalOutMax=[]  SumDenOutMin=[]  SumDenOutMax=[]  SumNumOutMin=[]  SumNumOutMax=[]  DivideOutMin=[]  DivideOutMax=[]  UdiffTsProdOutMin=[]  UdiffTsProdOutMax=[]  NTsProdOutMin=[]  NTsProdOutMax=[]  UintegralTsProdOutMin=[]  UintegralTsProdOutMax=[]  UngainTsProdOutMin=[]  UngainTsProdOutMax=[]  ClampingZeroOutDataTypeStr=Inherit: Inherit via back propagation  ClampingZeroOutMin=[]  ClampingZeroOutMax=[]  FilterDenConstantOutDataTypeStr=Inherit: Inherit via back propagation  FilterDenConstantOutMin=[]  FilterDenConstantOutMax=[]  PCopyOutDataTypeStr=Inherit: Inherit via back propagation  PCopyOutMin=[]  PCopyOutMax=[]  NCopyOutDataTypeStr=Inherit: Inherit via back propagation  NCopyOutMin=[]  NCopyOutMax=[]  IntegratorContinuousStateAttributes=''  IntegratorStateMustResolveToSignalObject=off  IntegratorRTWStateStorageClass=Auto  FilterContinuousStateAttributes=''  FilterStateMustResolveToSignalObject=off  FilterRTWStateStorageClass=Auto  ParallelPVariant=InternalParameters  IdealPVariant=Disabled  IVariant=InternalParameters  DVariant=InternalParameters  IntegratorVariant=Discrete  SatVariant=Enabled  AWVariant=DiscClampingParallel  PCopyVariant=Disabled  TRVariant=Disabled  FdbkBlocksVariant=Forward  IdealPFdbkVariant=Disabled  SatFdbkVariant=Disabled  DerivativeFilterVariant=Differentiator  NVariant=Passthrough  NCopyVariant=Disabled_SignalSpec  FilterICVariant=InternalICsDifferentiator  IntegratorICVariant=InternalICs  ExternalResetVariant=Disabled  TRSumVariant=Passthrough  SumFdbkVariant=Disabled  SumVariant=Sum_PID  TsampFilterVariant=ExternalTs  TsampNgainVariant=Passthrough  TsampIntegralVariant=ExternalTs  ExternalSaturationOutDataTypeStr=Inherit: Same as second input  DerivativeSourceVariant=ErrorSignal
  Product : Product  OutDataTypeStr=single
  Product1 : Product
  Subtract : Sum  Inputs=+-
  Subtract1 : Sum  Inputs=+-
  Elevator Cmd [rad] : Outport
  wires:
  Pitch Stick/1 -> Product/2
  Constant/1 -> Product/1
  Product/1 -> Angle Conversion/1
  Angle Conversion/1 -> Subtract/1
  Pitch Angle [rad]/1 -> Subtract/2
  PID Controller/1 -> Subtract1/1
  Product1/1 -> Subtract1/2
  Pitch Rate [rad/s]/1 -> Product1/1
  Constant1/1 -> Product1/2
  Subtract1/1 -> Elevator Cmd [rad]/1
  Constant2/1 -> PID Controller/2
  Subtract/1 -> PID Controller/1

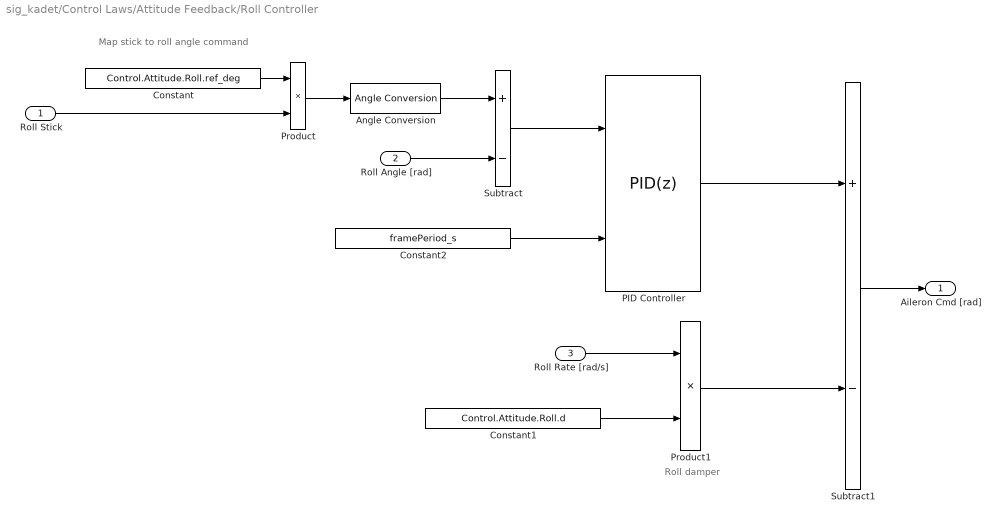
== system sig_kadet/Control Laws/Attitude Feedback/Roll Controller ==
  note: Map stick to roll angle command
  note: Roll damper
  Roll Stick : Inport
  Roll Angle [rad] : Inport  Port=2
  Roll Rate [rad/s] : Inport  Port=3
  Angle Conversion : aerolibconvert2/Angle Conversion  IU=deg  OU=rad
  Constant : Constant  Value=Control.Attitude.Roll.ref_deg  OutDataTypeStr=single
  Constant1 : Constant  Value=Control.Attitude.Roll.d  OutDataTypeStr=single
  Constant2 : Constant  Value=framePeriod_s  OutDataTypeStr=single
  PID Controller : slpidlib/PID Controller  Controller=PID  Form=Parallel  TimeDomain=Discrete-time  UseExternalTs=on  SampleTime=-1  IntegratorMethod=Forward Euler  FilterMethod=Forward Euler  ControllerParametersSource=internal  P=Control.Attitude.Roll.p  I=Control.Attitude.Roll.i  UseKiTs=off  D=0  UseExternalDerivativeSource=off  N=100  UseFilter=off  TunerSelectOption=Transfer Function Based (PID Tuner App)  ZeroCross=off  InitialConditionSource=internal  InitialConditionForIntegrator=0  InitialConditionForFilter=0  DifferentiatorICPrevScaledInput=0  ExternalReset=none  TrackingMode=off  Kt=1  LimitOutput=on  SatLimitsSource=internal  UpperSaturationLimit=deg2rad(Control.ail_lim_deg)  LowerSaturationLimit=-deg2rad(Control.ail_lim_deg)  LinearizeAsGain=on  AntiWindupMode=clamping  Kb=1  LimitIntegrator=off  UpperIntegratorSaturationLimit=inf  LowerIntegratorSaturationLimit=-inf  PGainOutDataTypeStr=single  PProdOutDataTypeStr=single  POutMin=[]  POutMax=[]  IGainOutDataTypeStr=single  IProdOutDataTypeStr=single  IOutMin=[]  IOutMax=[]  DGainOutDataTypeStr=single  DProdOutDataTypeStr=single  DOutMin=[]  DOutMax=[]  NOutMin=[]  NOutMax=[]  SumOutDataTypeStr=single  SumOutMin=[]  SumOutMax=[]  SaturationOutDataTypeStr=single  SaturationOutMin=[]  SaturationOutMax=[]  PParamMin=[]  PParamMax=[]  IParamMin=[]  IParamMax=[]  DParamMin=[]  DParamMax=[]  NParamMin=[]  NParamMax=[]  KbParamMin=[]  KbParamMax=[]  KtParamMin=[]  KtParamMax=[]  KbOutMin=[]  KbOutMax=[]  KtOutMin=[]  KtOutMax=[]  IntegratorOutMin=[]  IntegratorOutMax=[]  FilterOutMin=[]  FilterOutMax=[]  SumI1OutMin=[]  SumI1OutMax=[]  SumI2OutMin=[]  SumI2OutMax=[]  SumI3OutMin=[]  SumI3OutMax=[]  SumI4OutMin=[]  SumI4OutMax=[]  SumDOutMin=[]  SumDOutMax=[]  DifferentiatorOutMin=[]  DifferentiatorOutMax=[]  FilterDiffOutCoefMin=[]  FilterDiffOutCoefMax=[]  ReciprocalOutMin=[]  ReciprocalOutMax=[]  SumDenOutMin=[]  SumDenOutMax=[]  SumNumOutMin=[]  SumNumOutMax=[]  DivideOutMin=[]  DivideOutMax=[]  UdiffTsProdOutMin=[]  UdiffTsProdOutMax=[]  NTsProdOutMin=[]  NTsProdOutMax=[]  UintegralTsProdOutMin=[]  UintegralTsProdOutMax=[]  UngainTsProdOutMin=[]  UngainTsProdOutMax=[]  ClampingZeroOutDataTypeStr=Inherit: Inherit via back propagation  ClampingZeroOutMin=[]  ClampingZeroOutMax=[]  FilterDenConstantOutDataTypeStr=Inherit: Inherit via back propagation  FilterDenConstantOutMin=[]  FilterDenConstantOutMax=[]  PCopyOutDataTypeStr=Inherit: Inherit via back propagation  PCopyOutMin=[]  PCopyOutMax=[]  NCopyOutDataTypeStr=Inherit: Inherit via back propagation  NCopyOutMin=[]  NCopyOutMax=[]  IntegratorContinuousStateAttributes=''  IntegratorStateMustResolveToSignalObject=off  IntegratorRTWStateStorageClass=Auto  FilterContinuousStateAttributes=''  FilterStateMustResolveToSignalObject=off  FilterRTWStateStorageClass=Auto  ParallelPVariant=InternalParameters  IdealPVariant=Disabled  IVariant=InternalParameters  DVariant=InternalParameters  IntegratorVariant=Discrete  SatVariant=Enabled  AWVariant=DiscClampingParallel  PCopyVariant=Disabled  TRVariant=Disabled  FdbkBlocksVariant=Forward  IdealPFdbkVariant=Disabled  SatFdbkVariant=Disabled  DerivativeFilterVariant=Differentiator  NVariant=Passthrough  NCopyVariant=Disabled_SignalSpec  FilterICVariant=InternalICsDifferentiator  IntegratorICVariant=InternalICs  ExternalResetVariant=Disabled  TRSumVariant=Passthrough  SumFdbkVariant=Disabled  SumVariant=Sum_PID  TsampFilterVariant=ExternalTs  TsampNgainVariant=Passthrough  TsampIntegralVariant=ExternalTs  ExternalSaturationOutDataTypeStr=Inherit: Same as second input  DerivativeSourceVariant=ErrorSignal
  Product : Product  OutDataTypeStr=single
  Product1 : Product
  Subtract : Sum  Inputs=+-
  Subtract1 : Sum  Inputs=+-
  Aileron Cmd [rad] : Outport
  wires:
  Constant2/1 -> PID Controller/2
  Subtract1/1 -> Aileron Cmd [rad]/1
  Constant1/1 -> Product1/2
  Roll Rate [rad/s]/1 -> Product1/1
  Product1/1 -> Subtract1/2
  PID Controller/1 -> Subtract1/1
  Subtract/1 -> PID Controller/1
  Roll Angle [rad]/1 -> Subtract/2
  Angle Conversion/1 -> Subtract/1
  Product/1 -> Angle Conversion/1
  Constant/1 -> Product/1
  Roll Stick/1 -> Product/2

== system sig_kadet/Control Laws/Attitude Feedback/Yaw Damper ==
  Yaw Rate [rad/s] : Inport
  Discrete Transfer Fcn : DiscreteTransferFcn  Numerator=[-0.065 0.065]  Denominator=[1 -0.9608]
  Rudder Cmd [rad] : Outport
  wires:
  Discrete Transfer Fcn/1 -> Rudder Cmd [rad]/1
  Yaw Rate [rad/s]/1 -> Discrete Transfer Fcn/1

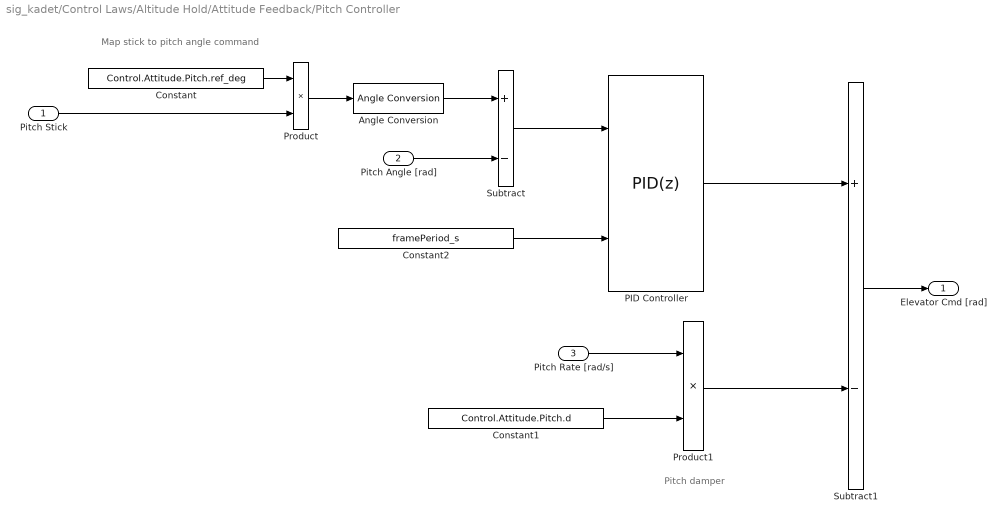
== system sig_kadet/Control Laws/Altitude Hold/Attitude Feedback/Pitch Controller ==
  note: Pitch damper
  note: Map stick to pitch angle command
  Pitch Stick : Inport
  Pitch Angle [rad] : Inport  Port=2
  Pitch Rate [rad/s] : Inport  Port=3
  Angle Conversion : aerolibconvert2/Angle Conversion  IU=deg  OU=rad
  Constant : Constant  Value=Control.Attitude.Pitch.ref_deg  OutDataTypeStr=single
  Constant1 : Constant  Value=Control.Attitude.Pitch.d  OutDataTypeStr=single
  Constant2 : Constant  Value=framePeriod_s  OutDataTypeStr=single
  PID Controller : slpidlib/PID Controller  Controller=PID  Form=Parallel  TimeDomain=Discrete-time  UseExternalTs=on  SampleTime=-1  IntegratorMethod=Forward Euler  FilterMethod=Forward Euler  ControllerParametersSource=internal  P=Control.Attitude.Pitch.p  I=Control.Attitude.Pitch.i  UseKiTs=off  D=0  UseExternalDerivativeSource=off  N=100  UseFilter=off  TunerSelectOption=Transfer Function Based (PID Tuner App)  ZeroCross=off  InitialConditionSource=internal  InitialConditionForIntegrator=0  InitialConditionForFilter=0  DifferentiatorICPrevScaledInput=0  ExternalReset=none  TrackingMode=off  Kt=1  LimitOutput=on  SatLimitsSource=internal  UpperSaturationLimit=deg2rad(Control.elev_lim_deg)  LowerSaturationLimit=-deg2rad(Control.elev_lim_deg)  LinearizeAsGain=on  AntiWindupMode=clamping  Kb=1  LimitIntegrator=off  UpperIntegratorSaturationLimit=inf  LowerIntegratorSaturationLimit=-inf  PGainOutDataTypeStr=single  PProdOutDataTypeStr=single  POutMin=[]  POutMax=[]  IGainOutDataTypeStr=single  IProdOutDataTypeStr=single  IOutMin=[]  IOutMax=[]  DGainOutDataTypeStr=single  DProdOutDataTypeStr=single  DOutMin=[]  DOutMax=[]  NOutMin=[]  NOutMax=[]  SumOutDataTypeStr=single  SumOutMin=[]  SumOutMax=[]  SaturationOutDataTypeStr=single  SaturationOutMin=[]  SaturationOutMax=[]  PParamMin=[]  PParamMax=[]  IParamMin=[]  IParamMax=[]  DParamMin=[]  DParamMax=[]  NParamMin=[]  NParamMax=[]  KbParamMin=[]  KbParamMax=[]  KtParamMin=[]  KtParamMax=[]  KbOutMin=[]  KbOutMax=[]  KtOutMin=[]  KtOutMax=[]  IntegratorOutMin=[]  IntegratorOutMax=[]  FilterOutMin=[]  FilterOutMax=[]  SumI1OutMin=[]  SumI1OutMax=[]  SumI2OutMin=[]  SumI2OutMax=[]  SumI3OutMin=[]  SumI3OutMax=[]  SumI4OutMin=[]  SumI4OutMax=[]  SumDOutMin=[]  SumDOutMax=[]  DifferentiatorOutMin=[]  DifferentiatorOutMax=[]  FilterDiffOutCoefMin=[]  FilterDiffOutCoefMax=[]  ReciprocalOutMin=[]  ReciprocalOutMax=[]  SumDenOutMin=[]  SumDenOutMax=[]  SumNumOutMin=[]  SumNumOutMax=[]  DivideOutMin=[]  DivideOutMax=[]  UdiffTsProdOutMin=[]  UdiffTsProdOutMax=[]  NTsProdOutMin=[]  NTsProdOutMax=[]  UintegralTsProdOutMin=[]  UintegralTsProdOutMax=[]  UngainTsProdOutMin=[]  UngainTsProdOutMax=[]  ClampingZeroOutDataTypeStr=Inherit: Inherit via back propagation  ClampingZeroOutMin=[]  ClampingZeroOutMax=[]  FilterDenConstantOutDataTypeStr=Inherit: Inherit via back propagation  FilterDenConstantOutMin=[]  FilterDenConstantOutMax=[]  PCopyOutDataTypeStr=Inherit: Inherit via back propagation  PCopyOutMin=[]  PCopyOutMax=[]  NCopyOutDataTypeStr=Inherit: Inherit via back propagation  NCopyOutMin=[]  NCopyOutMax=[]  IntegratorContinuousStateAttributes=''  IntegratorStateMustResolveToSignalObject=off  IntegratorRTWStateStorageClass=Auto  FilterContinuousStateAttributes=''  FilterStateMustResolveToSignalObject=off  FilterRTWStateStorageClass=Auto  ParallelPVariant=InternalParameters  IdealPVariant=Disabled  IVariant=InternalParameters  DVariant=InternalParameters  IntegratorVariant=Discrete  SatVariant=Enabled  AWVariant=DiscClampingParallel  PCopyVariant=Disabled  TRVariant=Disabled  FdbkBlocksVariant=Forward  IdealPFdbkVariant=Disabled  SatFdbkVariant=Disabled  DerivativeFilterVariant=Differentiator  NVariant=Passthrough  NCopyVariant=Disabled_SignalSpec  FilterICVariant=InternalICsDifferentiator  IntegratorICVariant=InternalICs  ExternalResetVariant=Disabled  TRSumVariant=Passthrough  SumFdbkVariant=Disabled  SumVariant=Sum_PID  TsampFilterVariant=ExternalTs  TsampNgainVariant=Passthrough  TsampIntegralVariant=ExternalTs  ExternalSaturationOutDataTypeStr=Inherit: Same as second input  DerivativeSourceVariant=ErrorSignal
  Product : Product  OutDataTypeStr=single
  Product1 : Product
  Subtract : Sum  Inputs=+-
  Subtract1 : Sum  Inputs=+-
  Elevator Cmd [rad] : Outport
  wires:
  Pitch Stick/1 -> Product/2
  Constant/1 -> Product/1
  Product/1 -> Angle Conversion/1
  Angle Conversion/1 -> Subtract/1
  Pitch Angle [rad]/1 -> Subtract/2
  Subtract/1 -> PID Controller/1
  PID Controller/1 -> Subtract1/1
  Product1/1 -> Subtract1/2
  Pitch Rate [rad/s]/1 -> Product1/1
  Constant1/1 -> Product1/2
  Subtract1/1 -> Elevator Cmd [rad]/1
  Constant2/1 -> PID Controller/2
